simulink model "test"  (R2023b)
settings: Solver=VariableStepAuto  StartTime=0.0  StopTime=0.2  RelTol=1e-3
values from neighbouring files (symbols this model uses):
  ext = Library_mtu_simulink_mtu_standard_parameters(ext)    [general_finger_MEE.m]
  ext_imr = Library_mtu_simulink_mtu_standard_parameters(ext_imr)    [index_middle_ring_finger_MEE.m]
  ext_small = Library_mtu_simulink_mtu_standard_parameters(ext_small)    [small_finger_MEE.m]
  ext_thumb = Library_mtu_simulink_mtu_standard_parameters(ext_thumb)    [thumb_MEE.m]
  flex = Library_mtu_simulink_mtu_standard_parameters(flex)    [general_finger_MEF.m]
  flex_imr = Library_mtu_simulink_mtu_standard_parameters(flex_imr)    [index_middle_ring_finger_MEF.m]
  flex_small = Library_mtu_simulink_mtu_standard_parameters(flex_small)    [small_finger_MEF.m]
  flex_thumb = Library_mtu_simulink_mtu_standard_parameters(flex_thumb)    [thumb_MEF.m]
undefined symbols (not defined in the file or in its folder): q, q2, X, Y, Z
libraries: sm_lib x147, Library_mtu_simulink x72, nesl_utility x55
(part 5 of 5)

== system test/Player2/index_ip9 ==
  In1 : Inport
  u [] : Inport  Port=2
  In3 : Inport  Port=3
  u []1 : Inport  Port=4
  ActivationDynamicsHatze : Library_mtu_simulink/ActivationDynamicsHatze  Act_Param=flex.ActDyn  Mus_Param=flex
  ActivationDynamicsHatze1 : Library_mtu_simulink/ActivationDynamicsHatze  Act_Param=ext.ActDyn  Mus_Param=ext
  MEE : Library_mtu_simulink/MuscleTendonUnit  Mus_Param=ext
  MEF : Library_mtu_simulink/MuscleTendonUnit  Mus_Param=flex
  PS-Simulink Converter1 : nesl_utility/PS-Simulink Converter  PhysicalDomain=network_engine_domain  SubClassName=ps_output  LeftPortType=input  RightPortType=output  PseudoPeriodic=off  Frequencies=[]  VectorFormat=1-D array  Unit=inherit  AffineConversion=off
  Scope : Scope
  Simulink-PS Converter1 : nesl_utility/Simulink-PS Converter  PhysicalDomain=network_engine_domain  SubClassName=ps_input  LeftPortType=input  RightPortType=output  PseudoPeriodic=off  Frequencies=[]  NoiseDistribution=none  NoiseParameters=[]  Unit=N*m  AffineConversion=off  FilteringAndDerivatives=provide  SimscapeFilterOrder=1  InputFilterTimeConstant=0.001  UdotUserProvided=0
  Sum : Sum  Inputs=+|+
  Sum1 : Sum  Inputs=+|+
  Sum2 : Sum  Inputs=-|-
  Terminator : Terminator
  Terminator1 : Terminator
  lmtcinit_MEE : Constant  Value=ext.l_MTC_init
  lmtcinit_MEF : Constant  Value=flex.l_MTC_init
  phi_dot : nesl_utility/PS-Simulink Converter  PhysicalDomain=network_engine_domain  SubClassName=ps_output  LeftPortType=input  RightPortType=output  PseudoPeriodic=off  Frequencies=[]  VectorFormat=1-D array  Unit=inherit  AffineConversion=off
  r_MEE*FMTU : Product
  r_MEE*phi : Product
  r_MEE*phidot : Product
  r_MEF*FMTU : Product
  r_MEF*phi : Product
  r_MEF*phidot : Product
  q : PMIOPort  Side=Left
  t : PMIOPort  Port=2  Side=Right
  w : PMIOPort  Port=3  Side=Left
  wires:
  MEE/3 -> Terminator1/1
  Sum2/1 -> Scope/1, Simulink-PS Converter1/1
  MEF/3 -> Terminator/1
  In3/1 -> r_MEE*FMTU/1, r_MEE*phi/2, r_MEE*phidot/2
  Sum/1 -> MEF/1
  ActivationDynamicsHatze1/1 -> MEE/3
  MEE/1 -> r_MEE*FMTU/2
  PS-Simulink Converter1/1 -> r_MEF*phi/1, r_MEE*phi/1
  ActivationDynamicsHatze/1 -> MEF/3
  In1/1 -> r_MEF*FMTU/1, r_MEF*phi/2, r_MEF*phidot/2
  r_MEE*phidot/1 -> MEE/2
  r_MEE*FMTU/1 -> Sum2/2
  MEF/1 -> r_MEF*FMTU/2
  r_MEF*phi/1 -> Sum/2
  r_MEF*FMTU/1 -> Sum2/1
  r_MEF*phidot/1 -> MEF/2
  MEE/2 -> ActivationDynamicsHatze1/2
  MEF/2 -> ActivationDynamicsHatze/2
  phi_dot/1 -> r_MEE*phidot/1, r_MEF*phidot/1
  Sum1/1 -> MEE/1
  lmtcinit_MEF/1 -> Sum/1
  lmtcinit_MEE/1 -> Sum1/1
  r_MEE*phi/1 -> Sum1/2
  u []1/1 -> ActivationDynamicsHatze1/1
  u []/1 -> ActivationDynamicsHatze/1
  connections:
  Simulink-PS Converter1/RConn1 -- t/RConn1
  PS-Simulink Converter1/LConn1 -- q/RConn1
  w/RConn1 -- phi_dot/LConn1
